simulink model "PSOBasedMPPTModel"  (R2016a)
settings: Solver=VariableStepAuto  SolverMode=SingleTasking  StartTime=0.0  StopTime=0.3  MaxStep=0.02  RelTol=1e-6
undefined symbols (not defined in the file or in its folder): sigbuilder_block
libraries: powerlib x11, re_lib x1
settings Model: Creator=abhidg.1  LastModifiedBy=staff
settings DebuggingCC: SFUnexpectedBacktrackingDiag=error  SFNoUnconditionalDefaultTransitionDiag=error
settings GRTTargetCC: TargetLangStandard=C99 (ISO)  GeneratePreprocessorConditionals=Use local settings
settings ConfigComp: CovMetricSettings=dwe  CovHtmlReporting=off  CovSaveCumulativeToWorkspaceVar=off  CovSaveSingleToWorkspaceVar=off  CovExternalEMLEnable=on

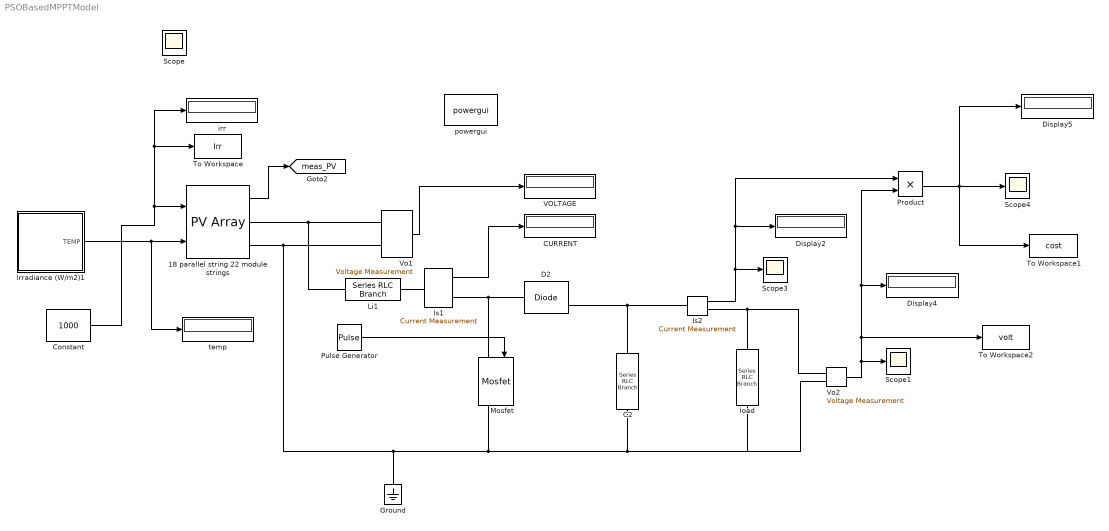
== system PSOBasedMPPTModel ==
  18 parallel string 22 module strings : re_lib/Solar/PV Array  Npar=1  Nser=1  PlotType=array @ 1000 W/m2 & specified temperatures  S_vec="[ 1000  500  1000 ]"  Temp_C_vec="[ 45 25  ]"  ModuleName=User-defined  PlotWhenSelected=on  Pm=100.44  Ncell=36  Voc=22.26  Isc=6.1  Vm=18  Im=5.58  beta_Voc_pc=-0.36099  alpha_Isc_pc=0.102  beta_Voc=-0.080356  alpha_Isc=0.006222  IL=6.1201  I0=2.2561e-10  nI=1.0037  Rsh=82.2528  Rs=0.27086  BAL=off  Tc=1e-6  Tfilter=5e-5
  C2 : powerlib/Elements/Series RLC Branch  LConnTagsString=__new0  RConnTagsString=__new0  BranchType=C  Resistance=1  Inductance=1e-3  SetiL0=off  InitialCurrent=0  Capacitance=220e-6  Setx0=off  InitialVoltage=0  Measurements=None
  CURRENT : Display
  Constant : Constant  Value=1000
  D2 : powerlib/Power Electronics/Diode  Ron=0.001  Lon=0  Vf=0.8  IC=0  UseSnubber=off  Rs=500  Cs=250e-9  Measurements=on
  Display2 : Display
  Display4 : Display
  Display5 : Display
  Ground : powerlib/Elements/Ground  LConnTagsString=a
  Irradiance (W/m2)1 : Subsystem  Tag=STV Subsys  LoadFcn=sigbuilder_block('load');  StartFcn=sigbuilder_block('start');  StopFcn=sigbuilder_block('stop');  ClipboardFcn=sigbuilder_block('clipboard');  mask(Sigbuilder block){}
      mask help: Sigbuilder GUI
      mask init:
      | if ~strcmp(get_param(bdroot(gcbh),'SimulationStatus'),'stopped') tuvar = sigbuilder_block('maskInit'); end
      settings: CopyFcn=sigbuilder_block('copy');  DeleteFcn=sigbuilder_block('delete');  ModelCloseFcn=sigbuilder_block('modelClose');  PreSaveFcn=sigbuilder_block('preSave');  PauseFcn=sigbuilder_block('pause')  ContinueFcn=sigbuilder_block('continue')  NameChangeFcn=sigbuilder_block('namechange');  OpenFcn=sigbuilder_block('open',[5.4 28.8 808.8 337.8 ]);  CloseFcn=sigbuilder_block('close');
      mask Display: plot(0,0,100,100,[10,10,40,40,10],[80,20,20,80,80],[40,10],[50,50], [40,27,10],[65,72,56],[40,25,25,10],[28,28,43,43]);
  Is1 : powerlib/Measurements/Current Measurement  PhasorSimulation=off  OutputType=Complex  PSBequivalent=0
  Is2 : powerlib/Measurements/Current Measurement  PhasorSimulation=off  OutputType=Complex  PSBequivalent=0
  Li1 : powerlib/Elements/Series RLC Branch  LConnTagsString=__new0  RConnTagsString=__new0  BranchType=L  Resistance=1  Inductance=1e-3  SetiL0=off  InitialCurrent=0  Capacitance=1e-6  Setx0=off  InitialVoltage=0  Measurements=None
  Mosfet : powerlib/Power Electronics/Mosfet  Ron=0.001  Lon=0  Rd=0.001  Vfd=0  IC=0  Rs=1e5  Cs=inf  Measurements=on
  Product : Product
  Pulse Generator : DiscretePulseGenerator  PulseType=Time based  Period=1/7000  PulseWidth=19
  Scope{,1,3..4} (4 alike) : Scope
  To Workspace : ToWorkspace  VariableName=Irr  SampleTime=-1
  To Workspace1 : ToWorkspace  VariableName=cost  SampleTime=-1
  To Workspace2 : ToWorkspace  VariableName=volt  SampleTime=-1
  VOLTAGE : Display
  Vo1 : powerlib/Measurements/Voltage Measurement  PhasorSimulation=off  OutputType=Complex  PSBequivalent=0
  Vo2 : powerlib/Measurements/Voltage Measurement  PhasorSimulation=off  OutputType=Complex  PSBequivalent=0
  irr : Display
  load : powerlib/Elements/Series RLC Branch  LConnTagsString=__new0  RConnTagsString=__new0  BranchType=R  Resistance=10  Inductance=1e-3  SetiL0=off  InitialCurrent=0  Capacitance=1e-6  Setx0=off  InitialVoltage=0  Measurements=None
  powergui : powerlib/powergui  Priority=1  SimulationMode=Continuous  SolverType=Tustin/Backward Euler (TBE)  SampleTime=50e-6  frequency=60  SPID=off  DisableSnubberDevices=off  DisableRonSwitches=off  DisableVfSwitches=off  SwTol=0  DisplayEquations=off  Interpol=off  ExternalGateDelay=off  methode=off  Ts=10  FunctionMessages=off  echomessages=off  HookPort=off  EnableUseOfTLC=off  x0status=blocks  frequencyindice=0  Pbase=100e6  ErrMax=1e-4  Iterations=50  UnitsV=kV  UnitsW=MW  buscounter=0  RestoreLinks=warning  ResistiveCurrentMeasurement=off  Frange=[0:2:500]  Ylog=off  Xlog=on  ShowGrid=off  save=off  variable=ZData  structure=0  ZoomFFT=off  StartTime=0.0  cycles=1  DisplayStyle=1  fundamental=60  FreqAxis=off  MaxFrequency=1000  frequencyindicesteady=1  RmsSteady=1  display=off
  temp : Display
  tag scope: meas_PV=global
  wires:
  Vo2/1 -> To Workspace2/1, Display4/1, Product/2, Scope1/1
  Pulse Generator/1 -> Mosfet/1
  Is2/1 -> Display2/1, Product/1, Scope3/1
  Product/1 -> To Workspace1/1, Display5/1, Scope4/1
  Is1/1 -> CURRENT/1
  Irradiance (W/m2)1/1(TEMP) -> temp/1, 18 parallel string 22 module strings/2
  18 parallel string 22 module strings/1 -> [meas_PV]
  Vo1/1 -> VOLTAGE/1
  Constant/1 -> To Workspace/1, irr/1, 18 parallel string 22 module strings/1
  connections:
  D2/RConn1 -- Is2/LConn1 -- C2/LConn1
  Is1/RConn1 -- Mosfet/LConn1 -- D2/LConn1
  Li1/RConn1 -- Is1/LConn1
  load/RConn1 -- Vo2/LConn1 -- Is2/RConn1
  18 parallel string 22 module strings/RConn2 -- Vo1/LConn2 -- Ground/LConn1 -- Mosfet/RConn1 -- Vo2/LConn2 -- load/LConn1 -- C2/RConn1
  Li1/LConn1 -- Vo1/LConn1 -- 18 parallel string 22 module strings/RConn1

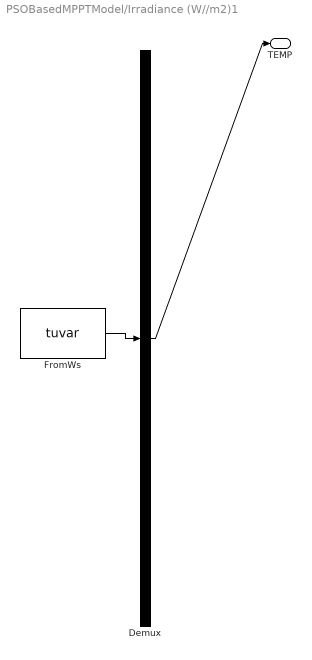
== system PSOBasedMPPTModel/Irradiance (W//m2)1 ==
  Demux : Demux  Tag=STV Demux  Outputs=1
  FromWs : FromWorkspace  Tag=STV FromWs  VariableName=tuvar  SampleTime=0
      SigBuilderData=|
      | common.afterFinalStr = 'Extrapolate'
      | common.sampleTime = '0'
      | dataSet.timeRange = [0 0.3]
      | dataSet.name = 'Sheet1'
      | sbobj.Name = 'Signal Builder'
      | sbobj.Groups.Name = 'Sheet1'
      | sbobj.Groups.Signals.Name = 'TEMP'
      | sbobj.Groups.Signals.XData = [0 0.3]
      | sbobj.Groups.Signals.YData = [22.5 22.5558510638]
      | sbobj.Groups.TimeRange = [0 0.3]
  TEMP : Outport  Tag=STV Outport
  wires:
  FromWs/1 -> Demux/1
  Demux/1 -> TEMP/1
